simulink model "FLC_PI_FUZZY_2"  (R2019b)
settings: Solver=VariableStepAuto  StartTime=0.0  StopTime=30  RelTol=1e-3
undefined symbols (not defined in the file or in its folder): sigbuilder_block
libraries: fuzblock x5
settings Model: Creator=Wero  LastModifiedBy=vsxrisi
settings DataIOCC: ReturnWorkspaceOutputs=off
settings DebuggingCC: ArithmeticOperatorsInVariantConditions=warning
settings SFSimCC: SimUseLocalCustomCode=off  CustomCodeUndefinedFunction=UseInterfaceOnly
settings RTWCC: RTWUseLocalCustomCode=off

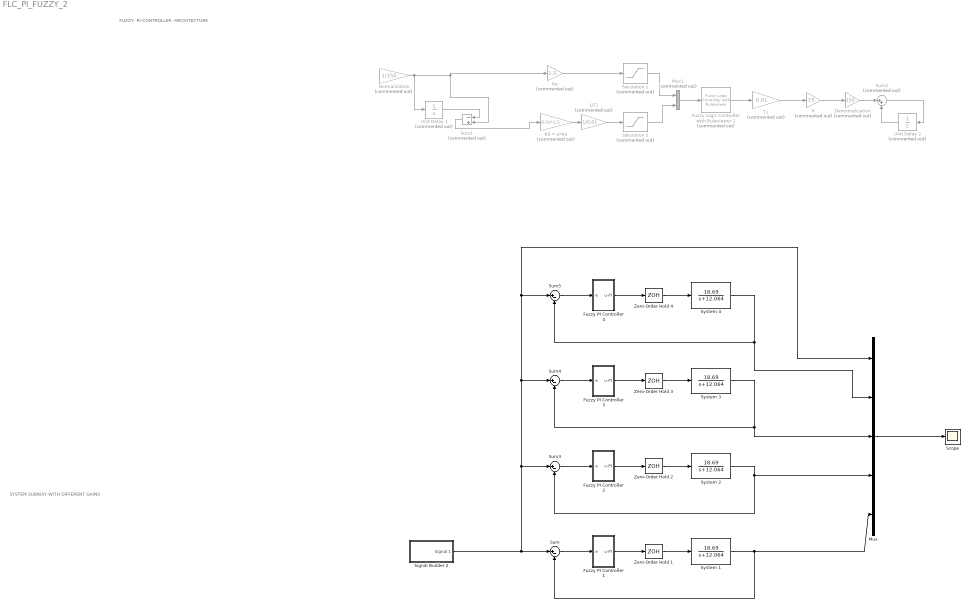
== system FLC_PI_FUZZY_2 ==
  note: FUZZY- PI-CONTROLLER -ARCHITECTURE
  note: SYSTEM SUBWAY WITH DIFFERENT GAINS
  1/T1 : Gain  Commented=on  Gain=1/0.01
  Denormalization : Gain  Commented=on  Gain=150
  Fuzzy Logic Controller with Ruleviewer 1 : fuzblock/Fuzzy Logic  Controller  with Ruleviewer  Commented=on  fismatrix=PIFuzzyController  Ts=0.01
  Fuzzy PI Controller 1 : Subsystem
  Fuzzy PI Controller 2 : Subsystem
  Fuzzy PI Controller 3 : Subsystem
  Fuzzy PI Controller 4 : Subsystem
  K : Gain  Commented=on  Gain=15
  Kd = a*Ke : Gain  Commented=on  Gain=0.03*1.5
  Ke : Gain  Commented=on  Gain=1.5
  Mux : Mux  Inputs=5
  Mux1 : Mux  Commented=on  Inputs=2
  Normalization : Gain  Commented=on  Gain=1/150
  Saturation 1 : Saturate  Commented=on
  Saturation 2 : Saturate  Commented=on
  "Scope " : Scope
  "Signal Builder 2 " : Subsystem  Tag=STV Subsys  LoadFcn=sigbuilder_block('load');  StartFcn=sigbuilder_block('start');  StopFcn=sigbuilder_block('stop');  ClipboardFcn=sigbuilder_block('clipboard');  mask(Sigbuilder block){tuvar=[0:10]}
      mask help: Simulink:masks:SigbuilderBlock_MD
      mask init:
      | if ~strcmp(get_param(bdroot(gcbh),'SimulationStatus'),'stopped') tuvar = sigbuilder_block('maskInit'); end
      settings: CopyFcn=sigbuilder_block('copy');  DeleteFcn=sigbuilder_block('delete');  ModelCloseFcn=sigbuilder_block('modelClose');  PreSaveFcn=sigbuilder_block('preSave');  PauseFcn=sigbuilder_block('pause');  ContinueFcn=sigbuilder_block('continue');  NameChangeFcn=sigbuilder_block('namechange');  OpenFcn=sigbuilder_block('open',[437.6 199.2 550.4 400 ]);  CloseFcn=sigbuilder_block('close');
      mask Display: plot(0, 0, 100, 100,[2, 2, 32, 32, 2], [68, 8, 8, 68, 68],[32, 2], [38, 38], [32, 19, 2],[53, 60, 44], [32, 17, 17, 2],[16, 16, 31, 31]);txt = getActiveGroup(gcbh);text(2, 100, txt,'verticalAlignment', 'top');
  Sum{,3..5} (4 alike) : Sum  Inputs=|+-
  Sum1 : Sum  Commented=on  Inputs=|-+
  Sum2 : Sum  Commented=on  Inputs=|++
  System {1..4} (4 alike) : TransferFcn  Numerator=[18.69]  Denominator=[1 12.064]
  T1 : Gain  Commented=on  Gain=0.01
  Unit Delay 1 : UnitDelay  Commented=on  SampleTime=-1  HasFrameUpgradeWarning=on
  Unit Delay 2 : UnitDelay  Commented=on  SampleTime=-1  HasFrameUpgradeWarning=on
  Zero-Order Hold {1..4} (4 alike) : ZeroOrderHold  SampleTime=-1
  wires:
  Zero-Order Hold 1/1 -> System 1/1
  System 1/1 -> Sum/2, Mux/5
  Mux/1 -> "Scope "/1
  Sum/1 -> Fuzzy PI Controller 1/1(e)
  Fuzzy PI Controller 1/1("u-PI ") -> Zero-Order Hold 1/1
  Saturation 2/1 -> Mux1/2
  Unit Delay 1/1 -> Sum1/1
  T1/1 -> K/1
  Denormalization/1 -> Sum2/1
  Ke/1 -> Saturation 1/1
  Saturation 1/1 -> Mux1/1
  Sum1/1 -> Kd = a*Ke/1
  Kd = a*Ke/1 -> 1/T1/1
  Normalization/1 -> Unit Delay 1/1, Sum1/2, Ke/1
  K/1 -> Denormalization/1
  Unit Delay 2/1 -> Sum2/2
  Sum2/1 -> Unit Delay 2/1
  Mux1/1 -> Fuzzy Logic Controller with Ruleviewer 1/1
  Fuzzy Logic Controller with Ruleviewer 1/1 -> T1/1
  1/T1/1 -> Saturation 2/1
  Sum3/1 -> Fuzzy PI Controller 2/1(e)
  System 2/1 -> Mux/4, Sum3/2
  Zero-Order Hold 2/1 -> System 2/1
  Fuzzy PI Controller 2/1("u-PI ") -> Zero-Order Hold 2/1
  Zero-Order Hold 3/1 -> System 3/1
  System 3/1 -> Mux/3, Sum4/2
  Fuzzy PI Controller 3/1("u-PI ") -> Zero-Order Hold 3/1
  Sum4/1 -> Fuzzy PI Controller 3/1(e)
  Zero-Order Hold 4/1 -> System 4/1
  Fuzzy PI Controller 4/1("u-PI ") -> Zero-Order Hold 4/1
  System 4/1 -> Mux/2, Sum5/2
  Sum5/1 -> Fuzzy PI Controller 4/1(e)
  "Signal Builder 2 "/1(Signal 1) -> Mux/1, Sum5/1, Sum4/1, Sum3/1, Sum/1

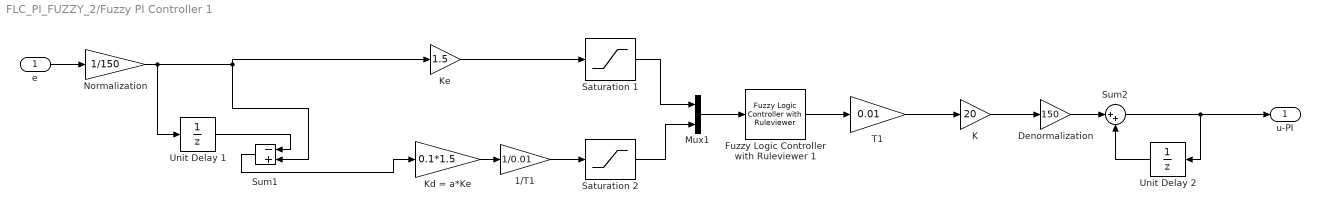
== system FLC_PI_FUZZY_2/Fuzzy PI Controller 1 ==
  e : Inport
  1/T1 : Gain  Gain=1/0.01
  Denormalization : Gain  Gain=150
  Fuzzy Logic Controller with Ruleviewer 1 : fuzblock/Fuzzy Logic  Controller  with Ruleviewer  fismatrix=PIFuzzyController  Ts=0.01
  K : Gain  Gain=20
  Kd = a*Ke : Gain  Gain=0.1*1.5
  Ke : Gain  Gain=1.5
  Mux1 : Mux  Inputs=2
  Normalization : Gain  Gain=1/150
  Saturation 1 : Saturate
  Saturation 2 : Saturate
  Sum1 : Sum  Inputs=|-+
  Sum2 : Sum  Inputs=|++
  T1 : Gain  Gain=0.01
  Unit Delay 1 : UnitDelay  SampleTime=-1  HasFrameUpgradeWarning=on
  Unit Delay 2 : UnitDelay  SampleTime=-1  HasFrameUpgradeWarning=on
  "u-PI " : Outport  VectorParamsAs1DForOutWhenUnconnected=off
  wires:
  1/T1/1 -> Saturation 2/1
  Saturation 2/1 -> Mux1/2
  Sum2/1 -> "u-PI "/1, Unit Delay 2/1
  Saturation 1/1 -> Mux1/1
  Mux1/1 -> Fuzzy Logic Controller with Ruleviewer 1/1
  Normalization/1 -> Unit Delay 1/1, Sum1/2, Ke/1
  Unit Delay 2/1 -> Sum2/2
  Fuzzy Logic Controller with Ruleviewer 1/1 -> T1/1
  Kd = a*Ke/1 -> 1/T1/1
  K/1 -> Denormalization/1
  Sum1/1 -> Kd = a*Ke/1
  e/1 -> Normalization/1
  T1/1 -> K/1
  Ke/1 -> Saturation 1/1
  Denormalization/1 -> Sum2/1
  Unit Delay 1/1 -> Sum1/1

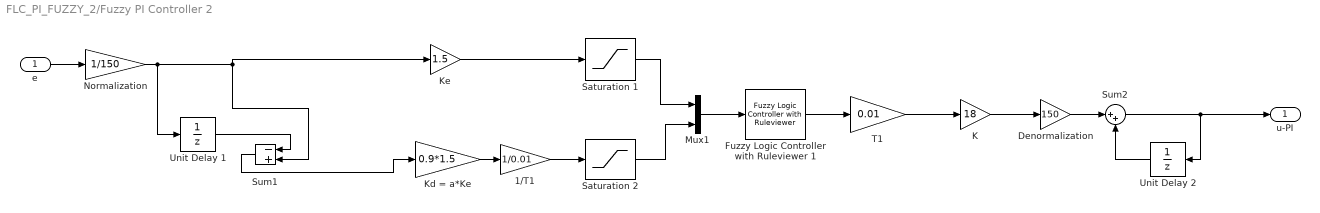
== system FLC_PI_FUZZY_2/Fuzzy PI Controller 2 ==
  e : Inport
  1/T1 : Gain  Gain=1/0.01
  Denormalization : Gain  Gain=150
  Fuzzy Logic Controller with Ruleviewer 1 : fuzblock/Fuzzy Logic  Controller  with Ruleviewer  fismatrix=PIFuzzyController  Ts=0.01
  K : Gain  Gain=18
  Kd = a*Ke : Gain  Gain=0.9*1.5
  Ke : Gain  Gain=1.5
  Mux1 : Mux  Inputs=2
  Normalization : Gain  Gain=1/150
  Saturation 1 : Saturate
  Saturation 2 : Saturate
  Sum1 : Sum  Inputs=|-+
  Sum2 : Sum  Inputs=|++
  T1 : Gain  Gain=0.01
  Unit Delay 1 : UnitDelay  SampleTime=-1  HasFrameUpgradeWarning=on
  Unit Delay 2 : UnitDelay  SampleTime=-1  HasFrameUpgradeWarning=on
  "u-PI " : Outport  VectorParamsAs1DForOutWhenUnconnected=off
  wires:
  1/T1/1 -> Saturation 2/1
  Saturation 2/1 -> Mux1/2
  Sum2/1 -> "u-PI "/1, Unit Delay 2/1
  Saturation 1/1 -> Mux1/1
  Mux1/1 -> Fuzzy Logic Controller with Ruleviewer 1/1
  Normalization/1 -> Unit Delay 1/1, Sum1/2, Ke/1
  Unit Delay 2/1 -> Sum2/2
  Fuzzy Logic Controller with Ruleviewer 1/1 -> T1/1
  Kd = a*Ke/1 -> 1/T1/1
  K/1 -> Denormalization/1
  Sum1/1 -> Kd = a*Ke/1
  e/1 -> Normalization/1
  T1/1 -> K/1
  Ke/1 -> Saturation 1/1
  Denormalization/1 -> Sum2/1
  Unit Delay 1/1 -> Sum1/1

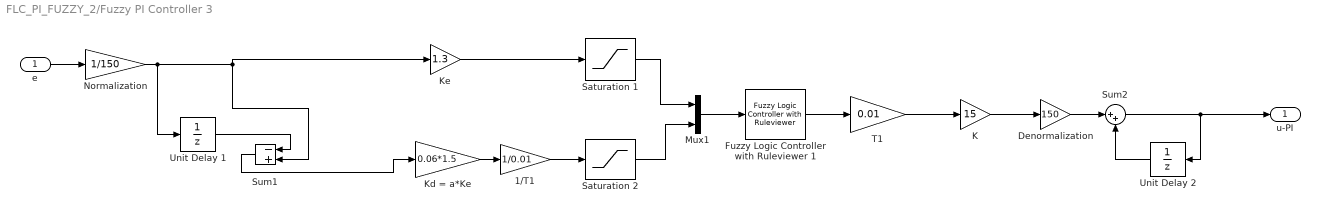
== system FLC_PI_FUZZY_2/Fuzzy PI Controller 3 ==
  e : Inport
  1/T1 : Gain  Gain=1/0.01
  Denormalization : Gain  Gain=150
  Fuzzy Logic Controller with Ruleviewer 1 : fuzblock/Fuzzy Logic  Controller  with Ruleviewer  fismatrix=PIFuzzyController  Ts=0.01
  K : Gain  Gain=15
  Kd = a*Ke : Gain  Gain=0.06*1.5
  Ke : Gain  Gain=1.3
  Mux1 : Mux  Inputs=2
  Normalization : Gain  Gain=1/150
  Saturation 1 : Saturate
  Saturation 2 : Saturate
  Sum1 : Sum  Inputs=|-+
  Sum2 : Sum  Inputs=|++
  T1 : Gain  Gain=0.01
  Unit Delay 1 : UnitDelay  SampleTime=-1  HasFrameUpgradeWarning=on
  Unit Delay 2 : UnitDelay  SampleTime=-1  HasFrameUpgradeWarning=on
  "u-PI " : Outport  VectorParamsAs1DForOutWhenUnconnected=off
  wires:
  1/T1/1 -> Saturation 2/1
  Saturation 2/1 -> Mux1/2
  Sum2/1 -> "u-PI "/1, Unit Delay 2/1
  Saturation 1/1 -> Mux1/1
  Mux1/1 -> Fuzzy Logic Controller with Ruleviewer 1/1
  Normalization/1 -> Unit Delay 1/1, Sum1/2, Ke/1
  Unit Delay 2/1 -> Sum2/2
  Fuzzy Logic Controller with Ruleviewer 1/1 -> T1/1
  Kd = a*Ke/1 -> 1/T1/1
  K/1 -> Denormalization/1
  Sum1/1 -> Kd = a*Ke/1
  e/1 -> Normalization/1
  T1/1 -> K/1
  Ke/1 -> Saturation 1/1
  Denormalization/1 -> Sum2/1
  Unit Delay 1/1 -> Sum1/1

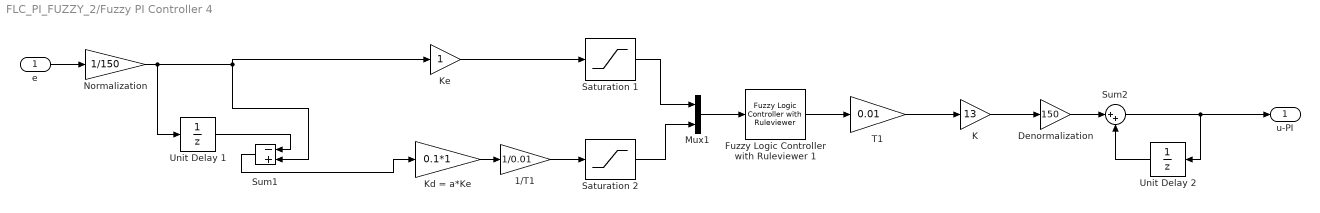
== system FLC_PI_FUZZY_2/Fuzzy PI Controller 4 ==
  e : Inport
  1/T1 : Gain  Gain=1/0.01
  Denormalization : Gain  Gain=150
  Fuzzy Logic Controller with Ruleviewer 1 : fuzblock/Fuzzy Logic  Controller  with Ruleviewer  fismatrix=PIFuzzyController  Ts=0.01
  K : Gain  Gain=13
  Kd = a*Ke : Gain  Gain=0.1*1
  Ke : Gain
  Mux1 : Mux  Inputs=2
  Normalization : Gain  Gain=1/150
  Saturation 1 : Saturate
  Saturation 2 : Saturate
  Sum1 : Sum  Inputs=|-+
  Sum2 : Sum  Inputs=|++
  T1 : Gain  Gain=0.01
  Unit Delay 1 : UnitDelay  SampleTime=-1  HasFrameUpgradeWarning=on
  Unit Delay 2 : UnitDelay  SampleTime=-1  HasFrameUpgradeWarning=on
  "u-PI " : Outport  VectorParamsAs1DForOutWhenUnconnected=off
  wires:
  1/T1/1 -> Saturation 2/1
  Saturation 2/1 -> Mux1/2
  Sum2/1 -> "u-PI "/1, Unit Delay 2/1
  Saturation 1/1 -> Mux1/1
  Mux1/1 -> Fuzzy Logic Controller with Ruleviewer 1/1
  Normalization/1 -> Unit Delay 1/1, Sum1/2, Ke/1
  Unit Delay 2/1 -> Sum2/2
  Fuzzy Logic Controller with Ruleviewer 1/1 -> T1/1
  Kd = a*Ke/1 -> 1/T1/1
  K/1 -> Denormalization/1
  Sum1/1 -> Kd = a*Ke/1
  e/1 -> Normalization/1
  T1/1 -> K/1
  Ke/1 -> Saturation 1/1
  Denormalization/1 -> Sum2/1
  Unit Delay 1/1 -> Sum1/1

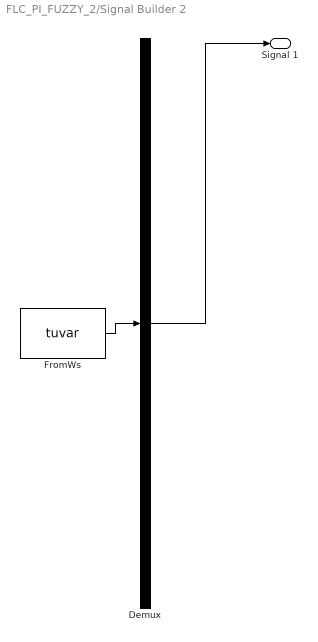
== system FLC_PI_FUZZY_2/Signal Builder 2  ==
  Demux : Demux  Tag=STV Demux  Outputs=1
  FromWs : FromWorkspace  Tag=STV FromWs  VariableName=tuvar  SampleTime=0
      SigBuilderData=|
      | common.afterFinalStr = 'Extrapolate'
      | common.sampleTime = 0
      | dataSet.timeRange = [0 30]
      | dataSet.name = 'Group 1'
      | sbobj.Groups.Name = 'Group 1'
      | sbobj.Groups.Signals.Name = 'Signal 1'
      | sbobj.Groups.Signals.XData = [0 10 20 30]
      | sbobj.Groups.Signals.YData = [0 150 150 0]
      | sbobj.Groups.TimeRange = [0 30]
  Signal 1 : Outport  Tag=STV Outport  VectorParamsAs1DForOutWhenUnconnected=off
  wires:
  Demux/1 -> Signal 1/1
  FromWs/1 -> Demux/1
